simulink model "amplant"  (R2021a)
settings: Solver=VariableStepAuto  StartTime=0.0  StopTime=10.0  RelTol=1e-3
settings Model: Creator=golam  LastModifiedBy=jamagola
settings SolverCC: AlgebraicLoopSolver=TrustRegion
settings DebuggingCC: SFMachineParentedDataDiag=warning

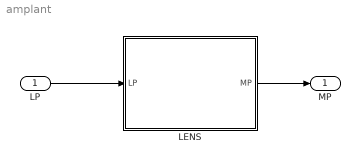
== system amplant ==
  LP : Inport
  LENS : Subsystem
  MP : Outport
  wires:
  LP/1 -> LENS/1(LP)
  LENS/1(MP) -> MP/1

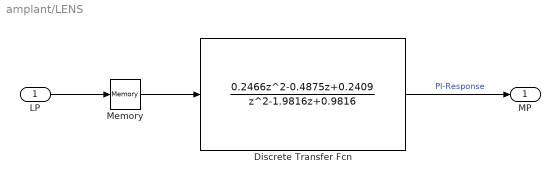
== system amplant/LENS ==
  LP : Inport
  Discrete Transfer Fcn : DiscreteTransferFcn  Numerator="[0.2466   -0.4875    0.2409]"  Denominator="[1.0000   -1.9816    0.9816]"  SampleTime=0.1
  Memory : Memory  InheritSampleTime=on  LinearizeAsDelay=on
  MP : Outport
  wires:
  Discrete Transfer Fcn/1 -> MP/1  "PI-Response"
  LP/1 -> Memory/1
  Memory/1 -> Discrete Transfer Fcn/1
